simulink model "z_MODEL_nieliniowy"  (R2020b)
settings: Solver=VariableStepAuto  StartTime=0.0  StopTime=210  RelTol=1e-3
values from neighbouring files (symbols this model uses):
  A = [ -0.01, 0; 0, -0.02]    [z_zadanie_inaczej.m]
  B = [1, 1; -0.25, 0.75]    [z_zadanie_inaczej.m]
  C = eye(2)    [z_zadanie_inaczej.m]
  c1 = 1    [z_zadanie_inaczej.m]
  c2 = 2    [z_zadanie_inaczej.m]
  F = Fa(:, 1:2)    [z_zadanie_inaczej.m]
  G2 = double(G2)    [z_zadanie_inaczej.m]
  K = 0.02    [z_zadanie_inaczej.m]
  M = Fa(:, 3:4)    [z_zadanie_inaczej.m]
  S = 1    [z_zadanie_inaczej.m]
undefined symbols (not defined in the file or in its folder): sigbuilder_block
settings Model: PauseTimes=0  Creator=Adam  LastModifiedBy=Adam

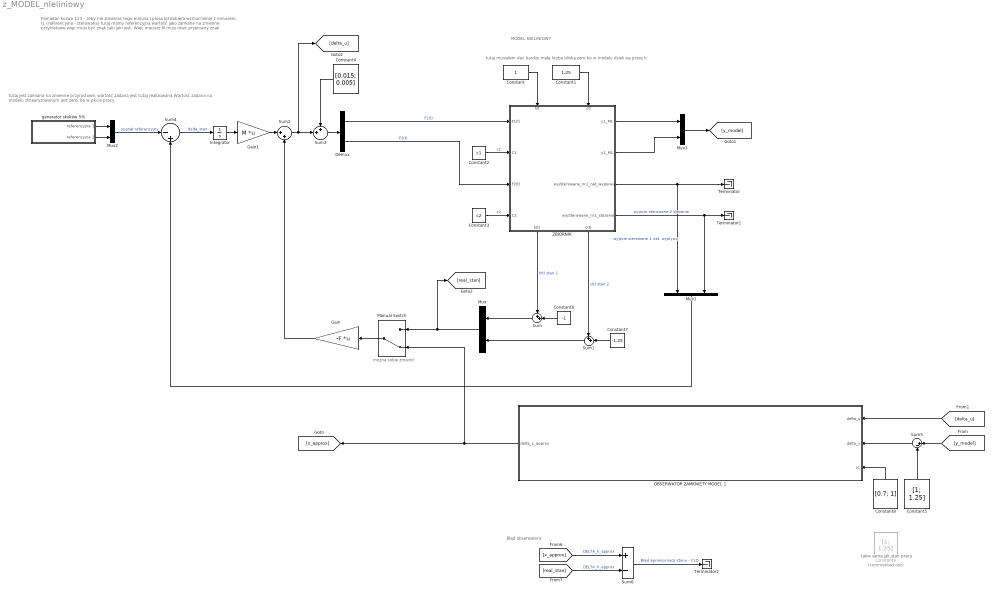
== system z_MODEL_nieliniowy ==
  note: Błąd obserwatora
  note: można sobie zmienić
  note: takie same jak stan pracy
  note: Pamietać kurwa 123 - żeby nie zmieniać tego minusa i plusa
      |
      | lqi dobiera wzmocnienie z minusem, tj. (referencyjna - sterowana) tutaj mamy referencyjną wartość jako zamiane na zmienne przyrostowe więc musi być znak taki jaki jest.
      | Więc macierz M musi mieć przeciwny znak
  note: tutaj jest zamiana na zmienne przyrostowe, wartość zadana jest tutaj realizowana
      | Wartość zadana na modelu zlinearyzowanym jest zero, bo w pkcie pracy.
  note: tutaj musiałem dać bardzo małą liczbe bliską zero bo w modelu dzieli się przez h
  note: MODEL NIELINIOWY
  Constant : Constant
  Constant1 : Constant  Value=1.25
  Constant2 : Constant  Value=c1
  Constant3 : Constant  Value=c2
  Constant4 : Constant  Value=[0.015; 0.005]  VectorParams1D=off
  Constant5 : Constant  Value=[1; 1.25]  VectorParams1D=off
  Constant6 : Constant  Value=-1
  Constant7 : Constant  Value=-1.25
  Constant8 : Constant  Value=[0.7; 1]  VectorParams1D=off
  Constant9 : Constant  Commented=on  Value=[1; 1.25]  VectorParams1D=off
  Demux : Demux  Outputs=2
  Gain : Gain  Gain=-F  Multiplication=Matrix(K*u) (u vector)
  Gain1 : Gain  Gain=M  Multiplication=Matrix(K*u) (u vector)
  Integrator : Integrator
  Manual Switch : ManualSwitch  CurrentSetting=0
  Mux{,1..3} (4 alike) : Mux  Inputs=2
  OBSERWATOR ZAMKNIĘTY MODEL 1 : Subsystem
  Sum : Sum  Inputs=++|
  Sum1 : Sum  Inputs=++|
  Sum2 : Sum  Inputs=|++
  Sum3 : Sum  Inputs=++|
  Sum4 : Sum  Inputs=|-+
  Sum5 : Sum  Inputs=|+-
  Sum6 : Sum  Inputs=+-
  Terminator : Terminator
  Terminator1 : Terminator
  Terminator2 : Terminator
  ZBIORNIK : Subsystem
      settings: PortSchema="{\"entries\":[{\"content\":{\"sides\":[{\"content\":{\"connectorIds\":[\"In1\",\"In2\",\"In3\",\"In4\"]},\"type\":\"ConnectorPlacement.EquallySpacedRectSide\",\"uuid\":\"d7534cdc-3a83-4663-9669-478cefb7ba54\"},{\"content\":{\"connectorIds\":[\"Out1\",\"Out2\",\"Out3\",\"Out4\"],\"side\":\"RIGHT\"},\"type\":\"ConnectorPlacement.EquallySpacedRectSide\",\"uuid\":\"43aa4112-be2a-4a64-a360-86159253405e\"},{\"content\":{\"connectorIds\":[\"In5\",\"In6\"],\"side\":\"TOP\"},\"type\":\"ConnectorPlacement.EquallySpacedRectSide\",\"uuid\":\"a87f647c-d073-49ff-8fa7-c7401791c269\"},{\"content\":{\"connectorIds\":[\"Out5\",\"Out6\"],\"side\":\"BOTTOM\"},\"type\":\"ConnectorPlacement.EquallySpacedRectSide\",\"uuid\":\"6d6aa66b-079d-45b1-a0b1-1cea6131b53f\"},{\"content\":{\"connectorIds\":[],\"side\":\"HIDDEN\"},\"type\":\"ConnectorPlacement.EquallySpacedRectSide\",\"uuid\":\"1d6cc66c-e8b9-4690-8052-ee4d3cbcc1b2\"}]},\"type\":\"ConnectorPlacement.EquallySpacedConnector\",\"uuid\":\"a7312018-d894-48d8-963b-edf04426afa5\"}],\"packageUris\":[\"http://schema.mathworks.com/mf0/Connector/R2020b\"],\"version\":\"1.0\"}"
  generator skoków 5% : Subsystem  Tag=STV Subsys  LoadFcn=sigbuilder_block('load');  StartFcn=sigbuilder_block('start');  StopFcn=sigbuilder_block('stop');  ClipboardFcn=sigbuilder_block('clipboard');  mask(Sigbuilder block){tuvar=[0:10]}
      mask help: Simulink:masks:SigbuilderBlock_MD
      mask init:
      | if ~strcmp(get_param(bdroot(gcbh),'SimulationStatus'),'stopped') tuvar = sigbuilder_block('maskInit'); end
      settings: CopyFcn=sigbuilder_block('copy');  DeleteFcn=sigbuilder_block('delete');  ModelCloseFcn=sigbuilder_block('modelClose');  PreSaveFcn=sigbuilder_block('preSave');  PauseFcn=sigbuilder_block('pause');  ContinueFcn=sigbuilder_block('continue');  NameChangeFcn=sigbuilder_block('namechange');  OpenFcn=sigbuilder_block('open',[409.8 142.2 550.8 400.2 ]);  CloseFcn=sigbuilder_block('close');
      mask Display: plot(0, 0, 100, 100,[2, 2, 32, 32, 2], [68, 8, 8, 68, 68],[32, 2], [38, 38], [32, 19, 2],[53, 60, 44], [32, 17, 17, 2],[16, 16, 31, 31]);txt = getActiveGroup(gcbh);text(2, 100, txt,'verticalAlignment', 'top');
  wires:
  Constant2/1 -> ZBIORNIK/2(C1)  "c1"
  Constant3/1 -> ZBIORNIK/4(C2)  "c2"
  Constant1/1 -> ZBIORNIK/6(c0)
  Constant/1 -> ZBIORNIK/5(h0)
  ZBIORNIK/5(h(t)) -> Sum/1  "h(t) stan 1"
  Constant6/1 -> Sum/2
  Constant7/1 -> Sum1/2
  ZBIORNIK/6(c(t)) -> Sum1/1  "c(t) stan 2"
  ZBIORNIK/3(wyjSterowane_nr1_nat_wyplywu) -> Mux1/1, Terminator/1  "wyjście sterowane 1 nat. wyplywu"
  ZBIORNIK/4(wyjSterowane_nr2_stezenie) -> Mux1/2, Terminator1/1  "wyjście sterowane 2 stezenie"
  Demux/1 -> ZBIORNIK/1(F1(t))  "F1(t)"
  Demux/2 -> ZBIORNIK/3(F2(t))  "F2(t)"
  Sum/1 -> Mux/1
  Sum1/1 -> Mux/2
  Mux/1 -> [real_stan], Manual Switch/1
  Gain/1 -> Sum2/2
  Gain1/1 -> Sum2/1
  Integrator/1 -> Gain1/1
  Sum2/1 -> [delta_u], Sum3/2
  Constant4/1 -> Sum3/1
  Sum3/1 -> Demux/1
  Sum4/1 -> Integrator/1  "delta_stan"
  Mux1/1 -> Sum4/2
  generator skoków 5%/1(referencyjna 1) -> Mux2/1
  generator skoków 5%/2(referencyjna 2) -> Mux2/2
  Mux2/1 -> Sum4/1  "sygnał referencyjny"
  ZBIORNIK/1(y1_M1) -> Mux3/1
  ZBIORNIK/2(y2_M1) -> Mux3/2
  Mux3/1 -> [y_model]
  [y_model] -> Sum5/1
  Constant5/1 -> Sum5/2
  Sum5/1 -> OBSERWATOR ZAMKNIĘTY MODEL 1/2(delta_y)
  OBSERWATOR ZAMKNIĘTY MODEL 1/1(delta_x_approx) -> [x_approx], Manual Switch/2
  [x_approx] -> Sum6/1  "DELTA_h_approx"
  [real_stan] -> Sum6/2  "DELTA_h_approx"
  Sum6/1 -> Terminator2/1  "Błąd aproksymacji stanu - CLO"
  [delta_u] -> OBSERWATOR ZAMKNIĘTY MODEL 1/1(delta_u)
  Constant8/1 -> OBSERWATOR ZAMKNIĘTY MODEL 1/3(IC)
  Manual Switch/1 -> Gain/1

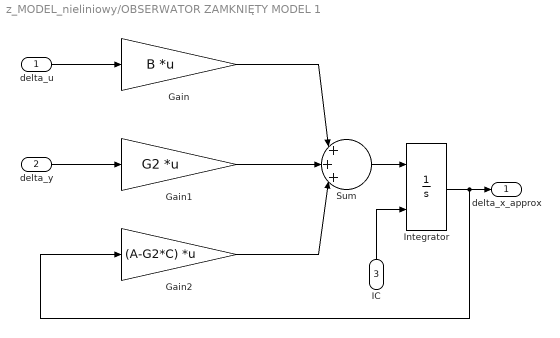
== system z_MODEL_nieliniowy/OBSERWATOR ZAMKNIĘTY MODEL 1 ==
  delta_u : Inport
  delta_y : Inport  Port=2
  IC : Inport  Port=3
  Gain : Gain  Gain=B  Multiplication=Matrix(K*u) (u vector)
  Gain1 : Gain  Gain=G2  Multiplication=Matrix(K*u) (u vector)
  Gain2 : Gain  Gain=(A-G2*C)  Multiplication=Matrix(K*u) (u vector)
  Integrator : Integrator  InitialConditionSource=external
  Sum : Sum  Inputs=|+++|
  delta_x_approx : Outport
  wires:
  Gain1/1 -> Sum/2
  Gain/1 -> Sum/1
  Gain2/1 -> Sum/3
  delta_u/1 -> Gain/1
  delta_y/1 -> Gain1/1
  Integrator/1 -> delta_x_approx/1, Gain2/1
  Sum/1 -> Integrator/1
  IC/1 -> Integrator/2

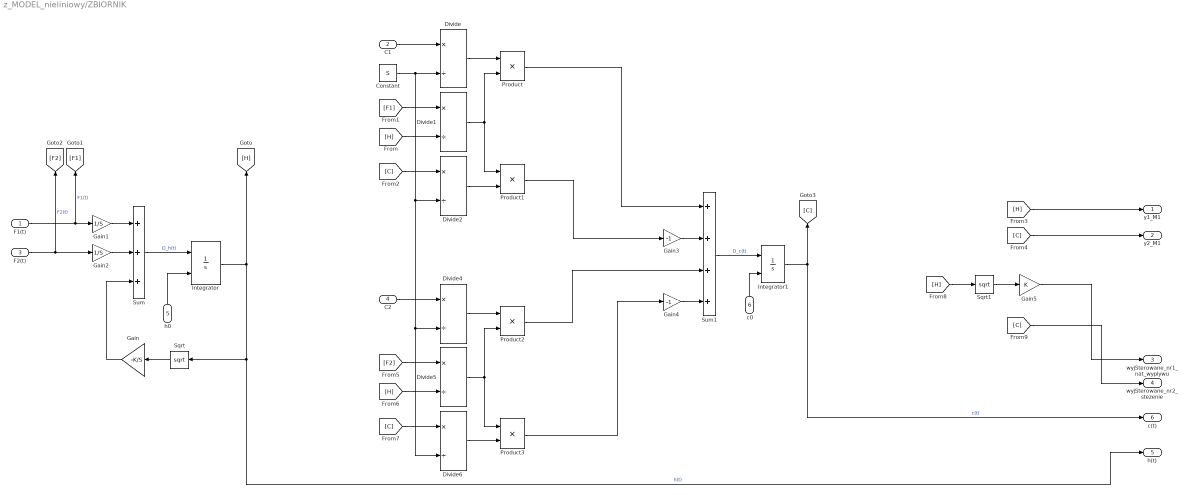
== system z_MODEL_nieliniowy/ZBIORNIK ==
  F1(t) : Inport
  C1 : Inport  Port=2
  F2(t) : Inport  Port=3
  C2 : Inport  Port=4
  h0 : Inport  Port=5
  c0 : Inport  Port=6
  Constant : Constant  Value=S
  Divide{,1..2,4..6} (6 alike) : Product  Inputs=*/
  Gain : Gain  Gain=-K/S
  Gain1 : Gain  Gain=1/S
  Gain2 : Gain  Gain=1/S
  Gain3 : Gain  Gain=-1
  Gain4 : Gain  Gain=-1
  Gain5 : Gain  Gain=K
  Integrator : Integrator  InitialConditionSource=external
  Integrator1 : Integrator  InitialConditionSource=external
  Product{,1..3} (4 alike) : Product
  Sqrt : Sqrt  OutputSignalType=real  SaturateOnIntegerOverflow=on
  Sqrt1 : Sqrt  SaturateOnIntegerOverflow=on
  Sum : Sum  Inputs=+++
  Sum1 : Sum  Inputs=++++
  y1_M1 : Outport
  y2_M1 : Outport  Port=2
  wyjSterowane_nr1_nat_wyplywu : Outport  Port=3
  wyjSterowane_nr2_stezenie : Outport  Port=4
  h(t) : Outport  Port=5
  c(t) : Outport  Port=6
  wires:
  C2/1 -> Divide4/1
  Product1/1 -> Gain3/1
  Product2/1 -> Sum1/3
  Divide5/1 -> Product3/1, Product2/2
  Gain4/1 -> Sum1/4
  [F2] -> Divide5/1
  Constant/1 -> Divide2/2, Divide4/2, Divide6/2, Divide/2
  C1/1 -> Divide/1
  Sum1/1 -> Integrator1/1  "D_c(t)"
  Product3/1 -> Gain4/1
  F1(t)/1 -> Gain1/1, [F1]  "F1(t)"
  [H] -> Divide1/2
  Gain1/1 -> Sum/1
  F2(t)/1 -> Gain2/1, [F2]  "F2(t)"
  Gain3/1 -> Sum1/2
  [C] -> Divide6/1
  Sum/1 -> Integrator/1  "D_h(t)"
  Divide4/1 -> Product2/1
  Sqrt/1 -> Gain/1
  Integrator1/1 -> [C], c(t)/1  "c(t)"
  Gain2/1 -> Sum/2
  Divide1/1 -> Product1/1, Product/2
  [C] -> Divide2/1
  [F1] -> Divide1/1
  [H] -> Divide5/2
  Divide6/1 -> Product3/2
  Divide/1 -> Product/1
  Product/1 -> Sum1/1
  h0/1 -> Integrator/2
  c0/1 -> Integrator1/2
  Divide2/1 -> Product1/2
  Integrator/1 -> Sqrt/1, h(t)/1, [H]  "h(t)"
  Gain/1 -> Sum/3
  [H] -> y1_M1/1
  [C] -> y2_M1/1
  Sqrt1/1 -> Gain5/1
  Gain5/1 -> wyjSterowane_nr1_nat_wyplywu/1
  [H] -> Sqrt1/1
  [C] -> wyjSterowane_nr2_stezenie/1

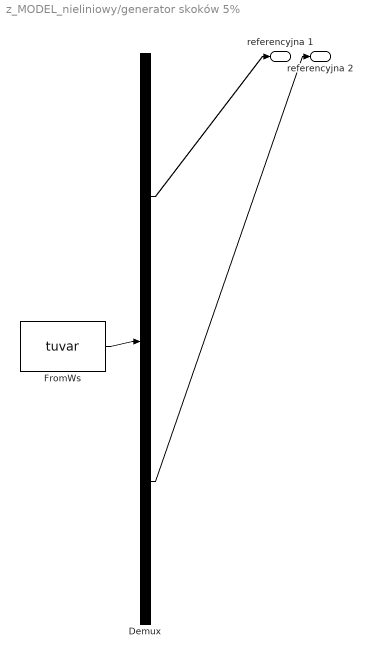
== system z_MODEL_nieliniowy/generator skoków 5% ==
  Demux : Demux  Tag=STV Demux  Outputs=2
      settings: DisplayOption=none
  FromWs : FromWorkspace  Tag=STV FromWs  VariableName=tuvar
      SigBuilderData=|
      | common.afterFinalStr = 'Extrapolate'
      | common.sampleTime = 0
      | dataSet.timeRange = [0 1000]
      | dataSet.name = 'skoki 5%'
      | sbobj.Groups.Name = 'skoki 5%'
      | sbobj.Groups.Signals(1).Name = 'referencyjna 1'
      | sbobj.Groups.Signals(1).XData = [0 60 60 110 110 160 160 210 210 1000]
      | sbobj.Groups.Signals(1).YData = [0.02 0.02 0.021 0.021 0.02 0.02 0.019 0.019 0.02 0.02]
      | sbobj.Groups.Signals(2).Name = 'referencyjna 2'
      | sbobj.Groups.Signals(2).XData = [0 60 60 110 110 160 160 210 210 1000]
      | sbobj.Groups.Signals(2).YData = [1.25 1.25 1.3125 1.3125 1.25 1.25 1.1875 1.1875 1.25 1.25]
      | sbobj.Groups.TimeRange = [0 1000]
  referencyjna 1 : Outport  Tag=STV Outport
  referencyjna 2 : Outport  Tag=STV Outport  Port=2
  wires:
  Demux/1 -> referencyjna 1/1
  Demux/2 -> referencyjna 2/1
  FromWs/1 -> Demux/1
